simulink model "rgfighter"  (Simulink 5.0)
settings: Solver=ode45  StartTime=0.0  StopTime=50.0  RelTol=1e-5
libraries: simulink x1

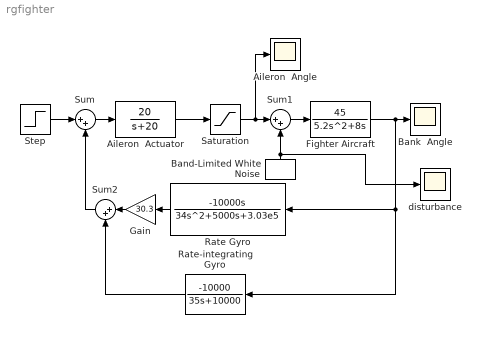
== system rgfighter ==
  Aileron  Actuator : TransferFcn  Numerator=20  Denominator=[1 20]
  Aileron  Angle : Scope
      settings: SaveName=dela  DataFormat=Array
  Band-Limited White Noise : simulink/Sources/Band-Limited White Noise  Orientation=up  Cov=[0.000001]  Ts=0.01  seed=[1000]
  Bank  Angle : Scope
      settings: SaveName=phi  DataFormat=Array  MaxDataPoints=15000
  Fighter Aircraft : TransferFcn  Numerator=[45]  Denominator=[5.2 8 0]
  Gain : Gain  Orientation=left  Gain=30.3  SaturateOnIntegerOverflow=on
  Rate Gyro : TransferFcn  Orientation=left  Numerator=[-10000 0]  Denominator=[34 5000 3.03e5]
  Rate-integrating Gyro : TransferFcn  Orientation=left  Numerator=-10000  Denominator=[35 10000]
  Saturation : Saturate  UpperLimit=0.087266  LowerLimit=-0.087266
  Step : Step  Time=0  After=0.349065850398866  SampleTime=0
  Sum : Sum  Inputs=|++  SaturateOnIntegerOverflow=on
  Sum1 : Sum  Inputs=|++  SaturateOnIntegerOverflow=on
  Sum2 : Sum  Orientation=left  Inputs=|++  SaturateOnIntegerOverflow=on
  disturbance : Scope
      settings: SaveName=d  DataFormat=Array  MaxDataPoints=15000
  wires:
  Sum1/1 -> Fighter Aircraft/1
  Band-Limited White Noise/1 -> Sum1/2, disturbance/1
  Fighter Aircraft/1 -> Bank  Angle/1, Rate Gyro/1, Rate-integrating Gyro/1
  Step/1 -> Sum/1
  Saturation/1 -> Sum1/1, Aileron  Angle/1
  Sum/1 -> Aileron  Actuator/1
  Aileron  Actuator/1 -> Saturation/1
  Rate Gyro/1 -> Gain/1
  Gain/1 -> Sum2/1
  Rate-integrating Gyro/1 -> Sum2/2
  Sum2/1 -> Sum/2
